simulink model "izaje_carro"  (R2019a)
settings: Solver=VariableStepAuto  StartTime=0.0  StopTime=10.0  RelTol=1e-3
undefined symbols (not defined in the file or in its folder): b_eqh, ih, J_eqh, Rd
settings Model: Creator=Adrián  LastModifiedBy=Adrián

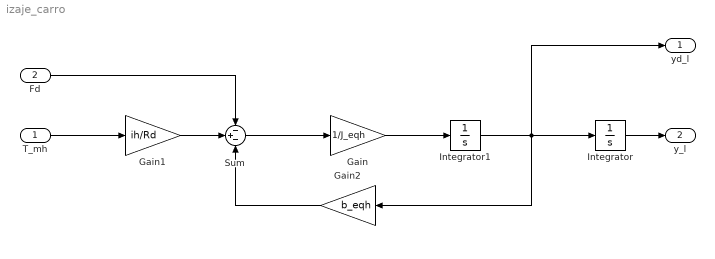
== system izaje_carro ==
  T_mh : Inport
  Fd : Inport  Port=2
  Gain : Gain  Gain=1/J_eqh
  Gain1 : Gain  Gain=ih/Rd
  Gain2 : Gain  Gain=b_eqh
  Integrator : Integrator
  Integrator1 : Integrator
  Sum : Sum  Inputs=-+-
  yd_l : Outport
  y_l : Outport  Port=2
  wires:
  Integrator1/1 -> Gain2/1, Integrator/1, yd_l/1
  Integrator/1 -> y_l/1
  Gain/1 -> Integrator1/1
  Sum/1 -> Gain/1
  Gain1/1 -> Sum/2
  T_mh/1 -> Gain1/1
  Fd/1 -> Sum/1
  Gain2/1 -> Sum/3
